simulink model "LAB4_PID"  (R2023a)
settings: Solver=VariableStepAuto  StartTime=0.0  StopTime=10.0  MaxStep=0.001  RelTol=1e-3
settings Model: Creator=alaam  LastModifiedBy=alaam

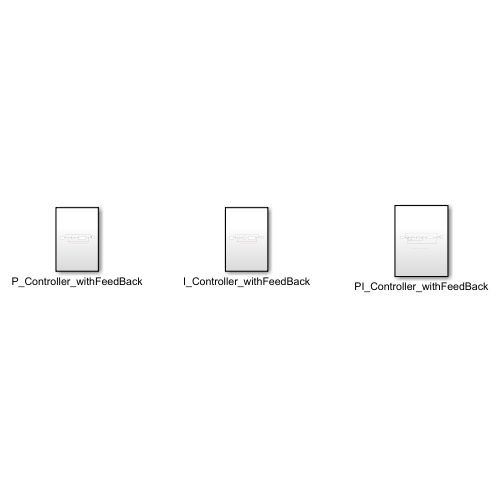
[thumbnail: Simulink's stored preview of the top-level diagram]
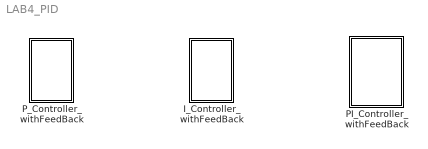
== system LAB4_PID ==
  I_Controller_withFeedBack : Subsystem
  PI_Controller_withFeedBack : Subsystem
  P_Controller_withFeedBack : Subsystem

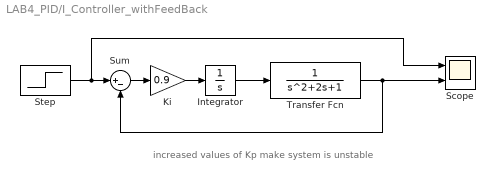
== system LAB4_PID/I_Controller_withFeedBack ==
  note: increased values of Kp make system is unstable
  Integrator : Integrator
  Ki : Gain  Gain=0.9
  Scope : Scope  NumInputPorts=2
  Step : Step  SampleTime=0
  Sum : Sum  Inputs=|+-
  Transfer Fcn : TransferFcn
  wires:
  Transfer Fcn/1 -> Sum/2, Scope/2
  Step/1 -> Scope/1, Sum/1
  Ki/1 -> Integrator/1
  Sum/1 -> Ki/1
  Integrator/1 -> Transfer Fcn/1

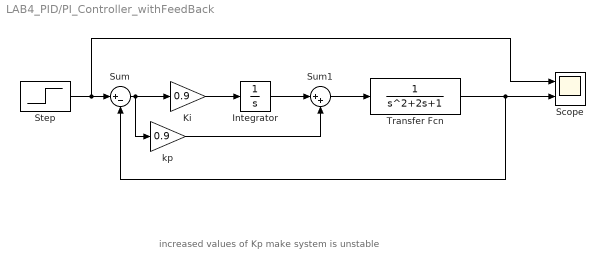
== system LAB4_PID/PI_Controller_withFeedBack ==
  note: increased values of Kp make system is unstable
  Integrator : Integrator
  Ki : Gain  Gain=0.9
  Scope : Scope  NumInputPorts=2
  Step : Step  SampleTime=0
  Sum : Sum  Inputs=|+-
  Sum1 : Sum  Inputs=|++
  Transfer Fcn : TransferFcn
  kp : Gain  Gain=0.9
  wires:
  Ki/1 -> Integrator/1
  Transfer Fcn/1 -> Sum/2, Scope/2
  Step/1 -> Scope/1, Sum/1
  Sum/1 -> kp/1, Ki/1
  Integrator/1 -> Sum1/1
  Sum1/1 -> Transfer Fcn/1
  kp/1 -> Sum1/2

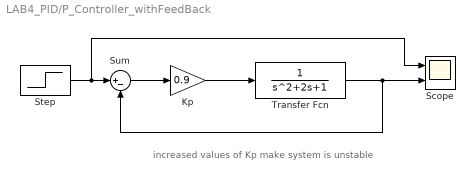
== system LAB4_PID/P_Controller_withFeedBack ==
  note: increased values of Kp make system is unstable
  Kp : Gain  Gain=0.9
  Scope : Scope  NumInputPorts=2
  Step : Step  SampleTime=0
  Sum : Sum  Inputs=|+-
  Transfer Fcn : TransferFcn
  wires:
  Sum/1 -> Kp/1
  Kp/1 -> Transfer Fcn/1
  Step/1 -> Scope/1, Sum/1
  Transfer Fcn/1 -> Sum/2, Scope/2
